simulink model "playground"  (R2024a)
settings: Solver=ode45  StartTime=0.0  StopTime=10.0  FixedStep=0.001  RelTol=1e-3
values from neighbouring files (symbols this model uses):
  a_r = 1.14 * 10^(-7)    (= 1.14e-07)    [start.m]    (also in startEnglPaper.m = 0.033; startReduced.m)
  a_rS = b    (= 0.033)    [startEnglPaper.m]
  A_x = 0.25    [playgrounMat.m]    (also in start.m; startEnglPaper.m; startReduced.m)
  A_y = 0.25    [playgrounMat.m]    (also in start.m; startEnglPaper.m; startReduced.m)
  A_z = 0.25    [playgrounMat.m]    (also in start.m; startEnglPaper.m; startReduced.m)
  b = 1.14 * 10^(-7)    (= 1.14e-07)    [start.m]    (also in startEnglPaper.m = 0.033; startReduced.m)
  g = 9.81    [playgrounMat.m]    (also in start.m; startEnglPaper.m; startReduced.m)
  gamma_d = pi/3    (= 1.0471975512)    [start.m]    (also in startReduced.m)
  I_r = 5.38 * 10 ^ (-5)    (= 5.38e-05)    [start.m]    (also in startEnglPaper.m = 3.38e-05; startReduced.m)
  I_x = 0.0151    [start.m]    (also in startEnglPaper.m = 0.004856; startReduced.m)
  I_y = 0.253    [start.m]    (also in startEnglPaper.m = 0.004856; startReduced.m)
  I_z = 0.0151    [start.m]    (also in startEnglPaper.m = 0.008801; startReduced.m)
  IrS = 5.38 * 10^(-5)    (= 5.38e-05)    [startEnglPaper.m]
  IxS = 0.0151    [startEnglPaper.m]
  IyS = IxS    (= 0.0151)    [startEnglPaper.m]
  IzS = 0.0253    [startEnglPaper.m]
  k = 1.045 * 10^(-11)    (= 1.045e-11)    [start.m]    (also in startEnglPaper.m = 2.98e-06; startReduced.m)
  K_gamma_D1 = K(1)    [playgrounMat.m]
  K_gamma_I1 = K(3)    [playgrounMat.m]
  K_gamma_P1 = K(2)    [playgrounMat.m]
  K_phi_D1 = 0.047    [startEnglPaper.m]
  K_phi_D11 = 0.093    [startEnglPaper.m]
  K_phi_D2 = 9.6    [startEnglPaper.m]
  K_phi_D22 = 19.2    [startEnglPaper.m]
  K_phi_DS = 0.14    [startEnglPaper.m]
  K_phi_I11 = 1.27    [startEnglPaper.m]
  K_phi_I22 = 262.144    [startEnglPaper.m]
  K_phi_P1 = 0.11    [startEnglPaper.m]
  K_phi_P11 = 0.5966    [startEnglPaper.m]
  K_phi_P2 = 23.04    [startEnglPaper.m]
  K_phi_P22 = 122.88    [startEnglPaper.m]
  K_phi_PS = 0.35    [startEnglPaper.m]
  K_psi_D = 40    [start.m]    (also in startEnglPaper.m = 9.6; startReduced.m)
  K_psi_D1 = 0.0844    [startEnglPaper.m]
  K_psi_D2 = 9.6    [startEnglPaper.m]
  K_psi_D22 = 19.2    [startEnglPaper.m]
  K_psi_DS = 0.24    [startEnglPaper.m]
  K_psi_I22 = 262.144    [startEnglPaper.m]
  K_psi_P = 143    [start.m]    (also in startEnglPaper.m = 23.04; startReduced.m)
  K_psi_P1 = 0.202    [startEnglPaper.m]
  K_psi_P2 = 23.04    [startEnglPaper.m]
  K_psi_P22 = 122.88    [startEnglPaper.m]
  K_psi_PS = 0.58    [startEnglPaper.m]
  K_theta_D = 58    [start.m]    (also in startEnglPaper.m = 9.6; startReduced.m)
  K_theta_D1 = 0.047    [startEnglPaper.m]
  K_theta_D2 = 9.6    [startEnglPaper.m]
  K_theta_D22 = 19.2    [startEnglPaper.m]
  K_theta_DS = 0.14    [startEnglPaper.m]
  K_theta_I22 = 262.144    [startEnglPaper.m]
  K_theta_P = 141    [start.m]    (also in startEnglPaper.m = 23.04; startReduced.m)
  K_theta_P1 = 0.11    [startEnglPaper.m]
  K_theta_P2 = 23.04    [startEnglPaper.m]
  K_theta_P22 = 122.88    [startEnglPaper.m]
  K_theta_PS = 0.35    [startEnglPaper.m]
  K_y_D = 13.58    [start.m]    (also in startReduced.m)
  K_y_P = 33.18    [start.m]    (also in startReduced.m)
  K_z_D1 = 4.42    [startEnglPaper.m]
  K_z_D2 = 4.42/m + A_z/m    (= 9.60905349794)    [startEnglPaper.m]
  K_z_DS = 13.58    [startEnglPaper.m]
  K_z_P1 = 11.2    [startEnglPaper.m]
  K_z_P2 = 11.2/m + A_z/m    (= 23.5596707819)    [startEnglPaper.m]
  K_z_PS = 33.18    [startEnglPaper.m]
  kl = 3 * 10^(-6)    (= 3e-06)    [startEnglPaper.m]
  l = 0.225    [start.m]    (also in startEnglPaper.m; startReduced.m)
  m = 1.44    [playgrounMat.m]    (also in start.m; startEnglPaper.m = 0.486; startReduced.m)
  m_s = [1/4 0 -1/(2*l) -1/(4*a_r); 1/4 -1/(2*l) 0 1/(4*a_r); 1/4 0 1/(2*l) -1/(4*a_r); 1/4 1/(2*l) 0 1/(4*a_r)]    [start.m]    (also in startReduced.m)
  mS = 1.44    [startEnglPaper.m]
  phi_d = 0.2    [startEnglPaper.m]
  phi_DesS = 0.2    [startEnglPaper.m]
  phi_init = 0    [startEnglPaper.m]
  phi_iS = 0;   deg2rad(10)    [startEnglPaper.m]
  psi_d = pi/5    (= 0.628318530718)    [start.m]    (also in startEnglPaper.m = 0.15; startReduced.m)
  psi_DesS = 0.15    [startEnglPaper.m]
  psi_init = 0    [startEnglPaper.m]
  psi_iS = 0    [startEnglPaper.m]
  theta_d = pi/4    (= 0.785398163397)    [start.m]    (also in startEnglPaper.m = 0.3; startReduced.m)
  theta_DesS = -0.1 * -3    (= 0.3)    [startEnglPaper.m]
  theta_init = 0    [startEnglPaper.m]
  theta_iS = 0    [startEnglPaper.m]
  x_init = 0    [startEnglPaper.m]
  x_iS = 0    [startEnglPaper.m]
  y_init = 0    [startEnglPaper.m]
  y_iS = 0    [startEnglPaper.m]
  z_d = 0.05 * 0    (= 0)    [startEnglPaper.m]
  z_DesS = 0.1    [startEnglPaper.m]
  z_init = 0    [startEnglPaper.m]
  z_iS = 0.0    (= 0)    [startEnglPaper.m]
undefined symbols (not defined in the file or in its folder): m_s_my
libraries: slpidlib x14
(part 1 of 4)
settings Model: Creator=Илья  LastModifiedBy=Илья

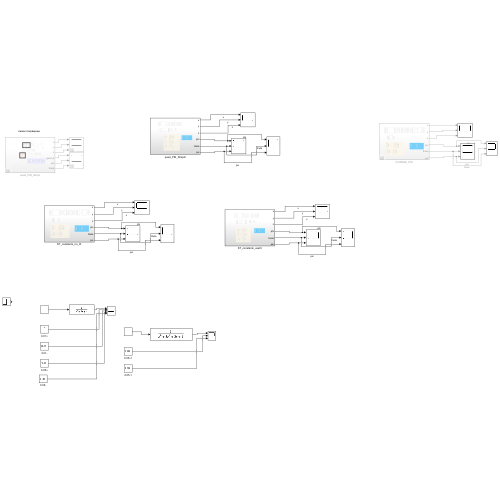
[thumbnail: Simulink's stored preview of the top-level diagram]
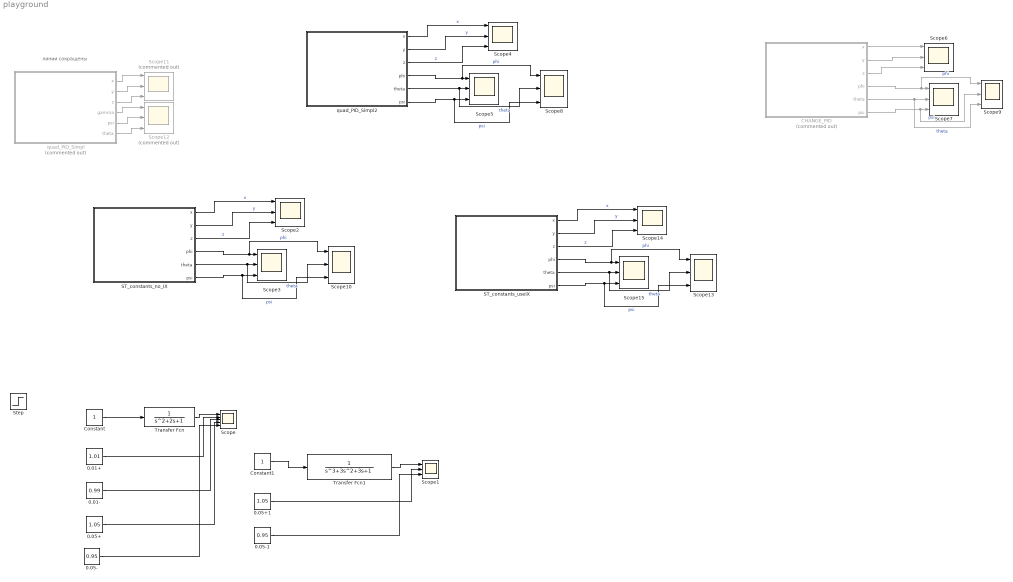
== system playground ==
  note: линии сокращены
  0.01+ : Constant  Value=1.01
  0.01- : Constant  Value=0.99
  0.05+ : Constant  Value=1.05
  0.05+1 : Constant  Value=1.05
  0.05- : Constant  Value=0.95
  0.05-1 : Constant  Value=0.95
  CHANGE_PID : Subsystem  Commented=on
  Constant : Constant
  Constant1 : Constant
  ST_constants_no_IX : Subsystem
  ST_constants_useIX : Subsystem
  Scope : Scope  NumInputPorts=5
  Scope{1..10,13..15} (13 alike) : Scope  NumInputPorts=3
  Scope11 : Scope  Commented=on  NumInputPorts=3
  Scope12 : Scope  Commented=on  NumInputPorts=3
  Step : Step  SampleTime=0
  Transfer Fcn : TransferFcn
  Transfer Fcn1 : TransferFcn  Denominator=[1 3 3 1]
  quad_PID_Simpl : Subsystem  Commented=on
  quad_PID_Simpl2 : Subsystem
  wires:
  Transfer Fcn/1 -> Scope/1
  Constant/1 -> Transfer Fcn/1
  0.01+/1 -> Scope/2
  0.01-/1 -> Scope/3
  0.05+/1 -> Scope/4
  0.05-/1 -> Scope/5
  Constant1/1 -> Transfer Fcn1/1
  Transfer Fcn1/1 -> Scope1/1
  0.05+1/1 -> Scope1/2
  0.05-1/1 -> Scope1/3
  quad_PID_Simpl/5(psi) -> Scope12/2
  quad_PID_Simpl/3(z) -> Scope11/3
  quad_PID_Simpl/4(gamma) -> Scope12/1
  quad_PID_Simpl/1(x) -> Scope11/1
  quad_PID_Simpl/2(y) -> Scope11/2
  quad_PID_Simpl/6(theta) -> Scope12/3
  quad_PID_Simpl2/2(y) -> Scope4/2  "y"
  quad_PID_Simpl2/3(z) -> Scope4/3  "z"
  quad_PID_Simpl2/6(psi) -> Scope8/3, Scope5/3  "psi"
  quad_PID_Simpl2/4(phi) -> Scope8/1, Scope5/1  "phi"
  quad_PID_Simpl2/5(theta) -> Scope8/2, Scope5/2  "theta"
  quad_PID_Simpl2/1(x) -> Scope4/1  "x"
  CHANGE_PID/1(x) -> Scope6/1
  CHANGE_PID/5(theta) -> Scope9/3, Scope7/2  "theta"
  CHANGE_PID/4(phi) -> Scope9/1, Scope7/1  "phi"
  CHANGE_PID/6(psi) -> Scope9/2, Scope7/3  "psi"
  CHANGE_PID/3(z) -> Scope6/3
  CHANGE_PID/2(y) -> Scope6/2
  ST_constants_no_IX/1(x) -> Scope2/1  "x"
  ST_constants_no_IX/5(theta) -> Scope3/2, Scope10/2  "theta"
  ST_constants_no_IX/4(phi) -> Scope3/1, Scope10/1  "phi"
  ST_constants_no_IX/6(psi) -> Scope3/3, Scope10/3  "psi"
  ST_constants_no_IX/3(z) -> Scope2/3  "z"
  ST_constants_no_IX/2(y) -> Scope2/2  "y"
  ST_constants_useIX/2(y) -> Scope14/2  "y"
  ST_constants_useIX/3(z) -> Scope14/3  "z"
  ST_constants_useIX/6(psi) -> Scope13/3, Scope15/3  "psi"
  ST_constants_useIX/4(phi) -> Scope13/1, Scope15/1  "phi"
  ST_constants_useIX/5(theta) -> Scope13/2, Scope15/2  "theta"
  ST_constants_useIX/1(x) -> Scope14/1  "x"

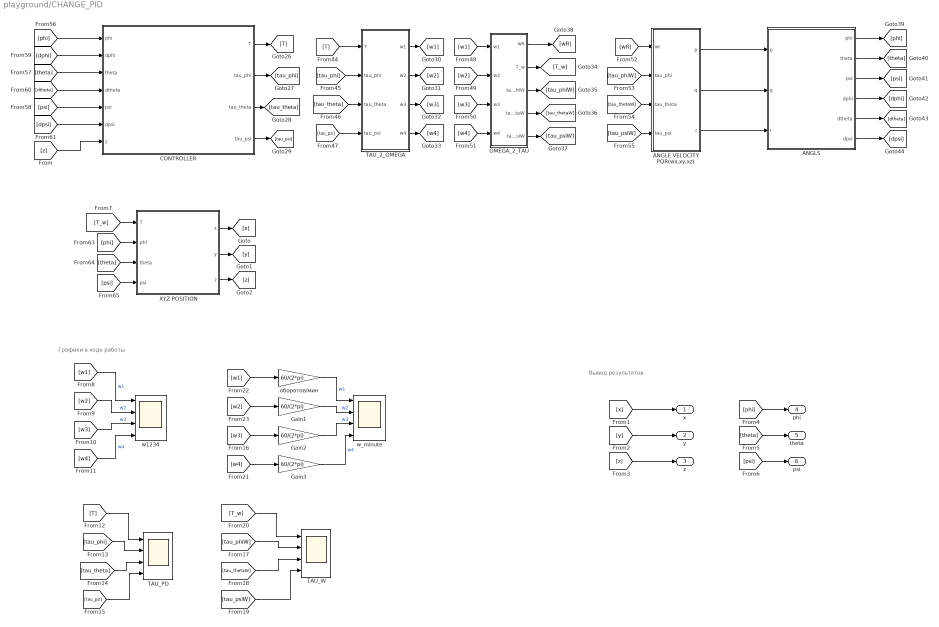
== system playground/CHANGE_PID ==
  note: Графики в ходе работы
  note: Вывод результатов
  ANGLE VELOCITY PQR(wx,xy,xz) : Subsystem
  ANGLS : Subsystem
  CONTROLLER : Subsystem
  Gain1 : Gain  Gain=60/(2*pi)
  Gain2 : Gain  Gain=60/(2*pi)
  Gain3 : Gain  Gain=60/(2*pi)
  OMEGA_2_TAU : Subsystem
  TAU_2_OMEGA : Subsystem
  TAU_PD : Scope  NumInputPorts=4
  TAU_W : Scope  NumInputPorts=4
  XYZ POSITION : Subsystem
  w1234 : Scope  NumInputPorts=4
  w_minute : Scope  NumInputPorts=4
  оборотов/мин : Gain  Gain=60/(2*pi)
  x : Outport
  y : Outport  Port=2
  z : Outport  Port=3
  phi : Outport  Port=4
  theta : Outport  Port=5
  psi : Outport  Port=6
  wires:
  Gain3/1 -> w_minute/4  "w4"
  Gain2/1 -> w_minute/3  "w3"
  Gain1/1 -> w_minute/2  "w2"
  оборотов/мин/1 -> w_minute/1  "w1"
  [w4] -> Gain3/1
  [w3] -> Gain2/1
  [w2] -> Gain1/1
  [w1] -> оборотов/мин/1
  [tau_psiW] -> TAU_W/4
  [tau_thetaW] -> TAU_W/3
  [tau_phiW] -> TAU_W/2
  [T_w] -> TAU_W/1
  [tau_psi] -> TAU_PD/4
  [tau_theta] -> TAU_PD/3
  [tau_phi] -> TAU_PD/2
  [T] -> TAU_PD/1
  [w4] -> w1234/4  "w4"
  [w3] -> w1234/3  "w3"
  [w2] -> w1234/2  "w2"
  [w1] -> w1234/1  "w1"
  [psi] -> psi/1
  [theta] -> theta/1
  [phi] -> phi/1
  [z] -> z/1
  [y] -> y/1
  [x] -> x/1
  [z] -> CONTROLLER/7(z)
  XYZ POSITION/3(z) -> [z]
  XYZ POSITION/2(y) -> [y]
  XYZ POSITION/1(x) -> [x]
  [psi] -> XYZ POSITION/4(psi)
  [theta] -> XYZ POSITION/3(theta)
  [phi] -> XYZ POSITION/2(phi)
  [T_w] -> XYZ POSITION/1(T)
  [psi] -> CONTROLLER/5(psi)
  [dpsi] -> CONTROLLER/6(dpsi)
  [dtheta] -> CONTROLLER/4(dtheta)
  [theta] -> CONTROLLER/3(theta)
  [dphi] -> CONTROLLER/2(dphi)
  [phi] -> CONTROLLER/1(phi)
  ANGLE VELOCITY PQR(wx,xy,xz)/3(r) -> ANGLS/3(r)
  ANGLE VELOCITY PQR(wx,xy,xz)/2(q) -> ANGLS/2(q)
  ANGLE VELOCITY PQR(wx,xy,xz)/1(p) -> ANGLS/1(p)
  ANGLS/6(dpsi) -> [dpsi]
  ANGLS/5(dtheta) -> [dtheta]
  ANGLS/4(dphi) -> [dphi]
  ANGLS/3(psi) -> [psi]
  ANGLS/2(theta) -> [theta]
  ANGLS/1(phi) -> [phi]
  [tau_psiW] -> ANGLE VELOCITY PQR(wx,xy,xz)/4(tau_psi)
  [tau_thetaW] -> ANGLE VELOCITY PQR(wx,xy,xz)/3(tau_theta)
  [tau_phiW] -> ANGLE VELOCITY PQR(wx,xy,xz)/2(tau_phi)
  [wR] -> ANGLE VELOCITY PQR(wx,xy,xz)/1(wr)
  OMEGA_2_TAU/1(wR) -> [wR]
  OMEGA_2_TAU/5(tau_psiW) -> [tau_psiW]
  OMEGA_2_TAU/4(tau_thetaW) -> [tau_thetaW]
  OMEGA_2_TAU/3(tau_phiW) -> [tau_phiW]
  OMEGA_2_TAU/2(T_w) -> [T_w]
  [w4] -> OMEGA_2_TAU/4(w4)
  [w3] -> OMEGA_2_TAU/3(w3)
  [w2] -> OMEGA_2_TAU/2(w2)
  [w1] -> OMEGA_2_TAU/1(w1)
  TAU_2_OMEGA/4(w4) -> [w4]
  TAU_2_OMEGA/3(w3) -> [w3]
  TAU_2_OMEGA/2(w2) -> [w2]
  TAU_2_OMEGA/1(w1) -> [w1]
  [tau_psi] -> TAU_2_OMEGA/4(tau_psi)
  [tau_theta] -> TAU_2_OMEGA/3(tau_theta)
  [tau_phi] -> TAU_2_OMEGA/2(tau_phi)
  [T] -> TAU_2_OMEGA/1(T)
  CONTROLLER/4(tau_psi) -> [tau_psi]
  CONTROLLER/3(tau_theta) -> [tau_theta]
  CONTROLLER/2(tau_phi) -> [tau_phi]
  CONTROLLER/1(T) -> [T]

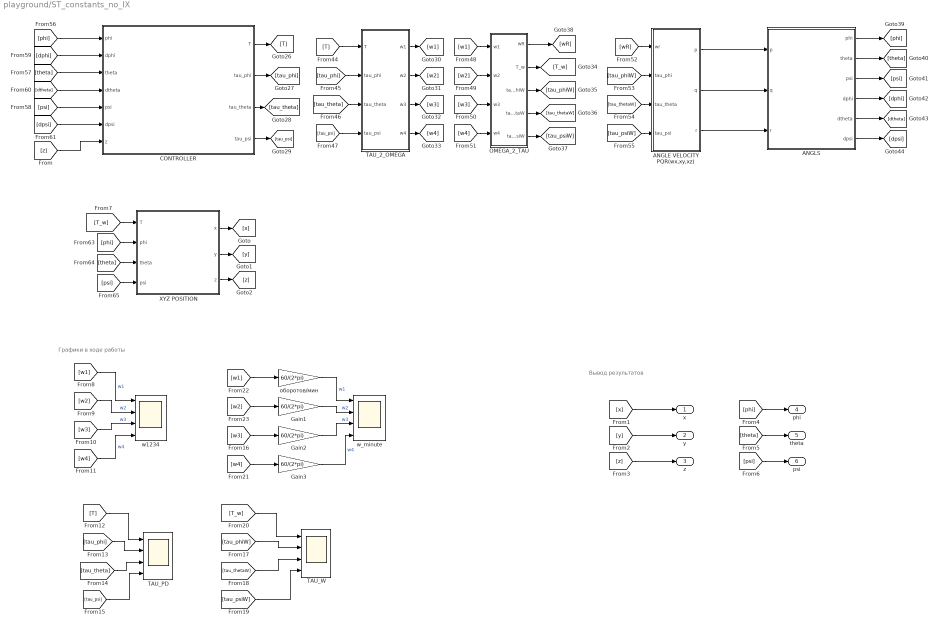
== system playground/ST_constants_no_IX ==
  note: Графики в ходе работы
  note: Вывод результатов
  ANGLE VELOCITY PQR(wx,xy,xz) : Subsystem
  ANGLS : Subsystem
  CONTROLLER : Subsystem
  Gain1 : Gain  Gain=60/(2*pi)
  Gain2 : Gain  Gain=60/(2*pi)
  Gain3 : Gain  Gain=60/(2*pi)
  OMEGA_2_TAU : Subsystem
  TAU_2_OMEGA : Subsystem
  TAU_PD : Scope  NumInputPorts=4
  TAU_W : Scope  NumInputPorts=4
  XYZ POSITION : Subsystem
  w1234 : Scope  NumInputPorts=4
  w_minute : Scope  NumInputPorts=4
  оборотов/мин : Gain  Gain=60/(2*pi)
  x : Outport
  y : Outport  Port=2
  z : Outport  Port=3
  phi : Outport  Port=4
  theta : Outport  Port=5
  psi : Outport  Port=6
  wires:
  Gain3/1 -> w_minute/4  "w4"
  Gain2/1 -> w_minute/3  "w3"
  Gain1/1 -> w_minute/2  "w2"
  оборотов/мин/1 -> w_minute/1  "w1"
  [w4] -> Gain3/1
  [w3] -> Gain2/1
  [w2] -> Gain1/1
  [w1] -> оборотов/мин/1
  [tau_psiW] -> TAU_W/4
  [tau_thetaW] -> TAU_W/3
  [tau_phiW] -> TAU_W/2
  [T_w] -> TAU_W/1
  [tau_psi] -> TAU_PD/4
  [tau_theta] -> TAU_PD/3
  [tau_phi] -> TAU_PD/2
  [T] -> TAU_PD/1
  [w4] -> w1234/4  "w4"
  [w3] -> w1234/3  "w3"
  [w2] -> w1234/2  "w2"
  [w1] -> w1234/1  "w1"
  [psi] -> psi/1
  [theta] -> theta/1
  [phi] -> phi/1
  [z] -> z/1
  [y] -> y/1
  [x] -> x/1
  [z] -> CONTROLLER/7(z)
  XYZ POSITION/3(z) -> [z]
  XYZ POSITION/2(y) -> [y]
  XYZ POSITION/1(x) -> [x]
  [psi] -> XYZ POSITION/4(psi)
  [theta] -> XYZ POSITION/3(theta)
  [phi] -> XYZ POSITION/2(phi)
  [T_w] -> XYZ POSITION/1(T)
  [psi] -> CONTROLLER/5(psi)
  [dpsi] -> CONTROLLER/6(dpsi)
  [dtheta] -> CONTROLLER/4(dtheta)
  [theta] -> CONTROLLER/3(theta)
  [dphi] -> CONTROLLER/2(dphi)
  [phi] -> CONTROLLER/1(phi)
  ANGLE VELOCITY PQR(wx,xy,xz)/3(r) -> ANGLS/3(r)
  ANGLE VELOCITY PQR(wx,xy,xz)/2(q) -> ANGLS/2(q)
  ANGLE VELOCITY PQR(wx,xy,xz)/1(p) -> ANGLS/1(p)
  ANGLS/6(dpsi) -> [dpsi]
  ANGLS/5(dtheta) -> [dtheta]
  ANGLS/4(dphi) -> [dphi]
  ANGLS/3(psi) -> [psi]
  ANGLS/2(theta) -> [theta]
  ANGLS/1(phi) -> [phi]
  [tau_psiW] -> ANGLE VELOCITY PQR(wx,xy,xz)/4(tau_psi)
  [tau_thetaW] -> ANGLE VELOCITY PQR(wx,xy,xz)/3(tau_theta)
  [tau_phiW] -> ANGLE VELOCITY PQR(wx,xy,xz)/2(tau_phi)
  [wR] -> ANGLE VELOCITY PQR(wx,xy,xz)/1(wr)
  OMEGA_2_TAU/1(wR) -> [wR]
  OMEGA_2_TAU/5(tau_psiW) -> [tau_psiW]
  OMEGA_2_TAU/4(tau_thetaW) -> [tau_thetaW]
  OMEGA_2_TAU/3(tau_phiW) -> [tau_phiW]
  OMEGA_2_TAU/2(T_w) -> [T_w]
  [w4] -> OMEGA_2_TAU/4(w4)
  [w3] -> OMEGA_2_TAU/3(w3)
  [w2] -> OMEGA_2_TAU/2(w2)
  [w1] -> OMEGA_2_TAU/1(w1)
  TAU_2_OMEGA/4(w4) -> [w4]
  TAU_2_OMEGA/3(w3) -> [w3]
  TAU_2_OMEGA/2(w2) -> [w2]
  TAU_2_OMEGA/1(w1) -> [w1]
  [tau_psi] -> TAU_2_OMEGA/4(tau_psi)
  [tau_theta] -> TAU_2_OMEGA/3(tau_theta)
  [tau_phi] -> TAU_2_OMEGA/2(tau_phi)
  [T] -> TAU_2_OMEGA/1(T)
  CONTROLLER/4(tau_psi) -> [tau_psi]
  CONTROLLER/3(tau_theta) -> [tau_theta]
  CONTROLLER/2(tau_phi) -> [tau_phi]
  CONTROLLER/1(T) -> [T]

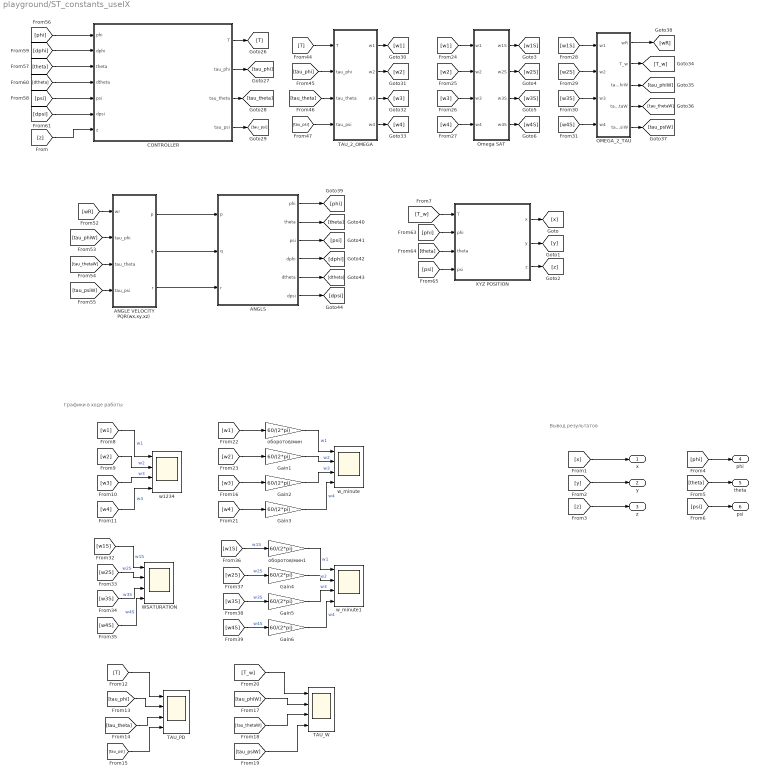
== system playground/ST_constants_useIX ==
  note: Вывод результатов
  note: Графики в ходе работы
  ANGLE VELOCITY PQR(wx,xy,xz) : Subsystem
  ANGLS : Subsystem
  CONTROLLER : Subsystem
  Gain{1..6} (6 alike) : Gain  Gain=60/(2*pi)
  OMEGA_2_TAU : Subsystem
  Omega SAT : Subsystem
  TAU_2_OMEGA : Subsystem
  TAU_PD : Scope  NumInputPorts=4
  TAU_W : Scope  NumInputPorts=4
  WSATURATION : Scope  NumInputPorts=4
  XYZ POSITION : Subsystem
  w1234 : Scope  NumInputPorts=4
  w_minute : Scope  NumInputPorts=4
  w_minute1 : Scope  NumInputPorts=4
  оборотов/мин : Gain  Gain=60/(2*pi)
  оборотов/мин1 : Gain  Gain=60/(2*pi)
  x : Outport
  y : Outport  Port=2
  z : Outport  Port=3
  phi : Outport  Port=4
  theta : Outport  Port=5
  psi : Outport  Port=6
  wires:
  CONTROLLER/1(T) -> [T]
  CONTROLLER/2(tau_phi) -> [tau_phi]
  CONTROLLER/3(tau_theta) -> [tau_theta]
  CONTROLLER/4(tau_psi) -> [tau_psi]
  [T] -> TAU_2_OMEGA/1(T)
  [tau_phi] -> TAU_2_OMEGA/2(tau_phi)
  [tau_theta] -> TAU_2_OMEGA/3(tau_theta)
  [tau_psi] -> TAU_2_OMEGA/4(tau_psi)
  TAU_2_OMEGA/1(w1) -> [w1]
  TAU_2_OMEGA/2(w2) -> [w2]
  TAU_2_OMEGA/3(w3) -> [w3]
  TAU_2_OMEGA/4(w4) -> [w4]
  [w1S] -> OMEGA_2_TAU/1(w1)
  [w2S] -> OMEGA_2_TAU/2(w2)
  [w3S] -> OMEGA_2_TAU/3(w3)
  [w4S] -> OMEGA_2_TAU/4(w4)
  OMEGA_2_TAU/2(T_w) -> [T_w]
  OMEGA_2_TAU/3(tau_phiW) -> [tau_phiW]
  OMEGA_2_TAU/4(tau_thetaW) -> [tau_thetaW]
  OMEGA_2_TAU/5(tau_psiW) -> [tau_psiW]
  OMEGA_2_TAU/1(wR) -> [wR]
  [wR] -> ANGLE VELOCITY PQR(wx,xy,xz)/1(wr)
  [tau_phiW] -> ANGLE VELOCITY PQR(wx,xy,xz)/2(tau_phi)
  [tau_thetaW] -> ANGLE VELOCITY PQR(wx,xy,xz)/3(tau_theta)
  [tau_psiW] -> ANGLE VELOCITY PQR(wx,xy,xz)/4(tau_psi)
  ANGLS/1(phi) -> [phi]
  ANGLS/2(theta) -> [theta]
  ANGLS/3(psi) -> [psi]
  ANGLS/4(dphi) -> [dphi]
  ANGLS/5(dtheta) -> [dtheta]
  ANGLS/6(dpsi) -> [dpsi]
  ANGLE VELOCITY PQR(wx,xy,xz)/1(p) -> ANGLS/1(p)
  ANGLE VELOCITY PQR(wx,xy,xz)/2(q) -> ANGLS/2(q)
  ANGLE VELOCITY PQR(wx,xy,xz)/3(r) -> ANGLS/3(r)
  [phi] -> CONTROLLER/1(phi)
  [dphi] -> CONTROLLER/2(dphi)
  [theta] -> CONTROLLER/3(theta)
  [dtheta] -> CONTROLLER/4(dtheta)
  [dpsi] -> CONTROLLER/6(dpsi)
  [psi] -> CONTROLLER/5(psi)
  [T_w] -> XYZ POSITION/1(T)
  [phi] -> XYZ POSITION/2(phi)
  [theta] -> XYZ POSITION/3(theta)
  [psi] -> XYZ POSITION/4(psi)
  XYZ POSITION/1(x) -> [x]
  XYZ POSITION/2(y) -> [y]
  XYZ POSITION/3(z) -> [z]
  [z] -> CONTROLLER/7(z)
  [x] -> x/1
  [y] -> y/1
  [z] -> z/1
  [phi] -> phi/1
  [theta] -> theta/1
  [psi] -> psi/1
  [w1] -> w1234/1  "w1"
  [w2] -> w1234/2  "w2"
  [w3] -> w1234/3  "w3"
  [w4] -> w1234/4  "w4"
  [T] -> TAU_PD/1
  [tau_phi] -> TAU_PD/2
  [tau_theta] -> TAU_PD/3
  [tau_psi] -> TAU_PD/4
  [T_w] -> TAU_W/1
  [tau_phiW] -> TAU_W/2
  [tau_thetaW] -> TAU_W/3
  [tau_psiW] -> TAU_W/4
  [w1] -> оборотов/мин/1
  [w2] -> Gain1/1
  [w3] -> Gain2/1
  [w4] -> Gain3/1
  оборотов/мин/1 -> w_minute/1  "w1"
  Gain1/1 -> w_minute/2  "w2"
  Gain2/1 -> w_minute/3  "w3"
  Gain3/1 -> w_minute/4  "w4"
  [w4] -> Omega SAT/4(w4)
  Omega SAT/2(w2S) -> [w2S]
  [w1] -> Omega SAT/1(w1)
  [w3] -> Omega SAT/3(w3)
  Omega SAT/4(w4S) -> [w4S]
  Omega SAT/1(w1S) -> [w1S]
  Omega SAT/3(w3S) -> [w3S]
  [w2] -> Omega SAT/2(w2)
  [w3S] -> Gain5/1  "w3S"
  Gain5/1 -> w_minute1/3  "w3"
  оборотов/мин1/1 -> w_minute1/1  "w1"
  [w4S] -> WSATURATION/4  "w4S"
  [w4S] -> Gain6/1  "w4S"
  [w1S] -> оборотов/мин1/1  "w1S"
  Gain6/1 -> w_minute1/4  "w4"
  Gain4/1 -> w_minute1/2  "w2"
  [w2S] -> WSATURATION/2  "w2S"
  [w3S] -> WSATURATION/3  "w3S"
  [w1S] -> WSATURATION/1  "w1S"
  [w2S] -> Gain4/1  "w2S"

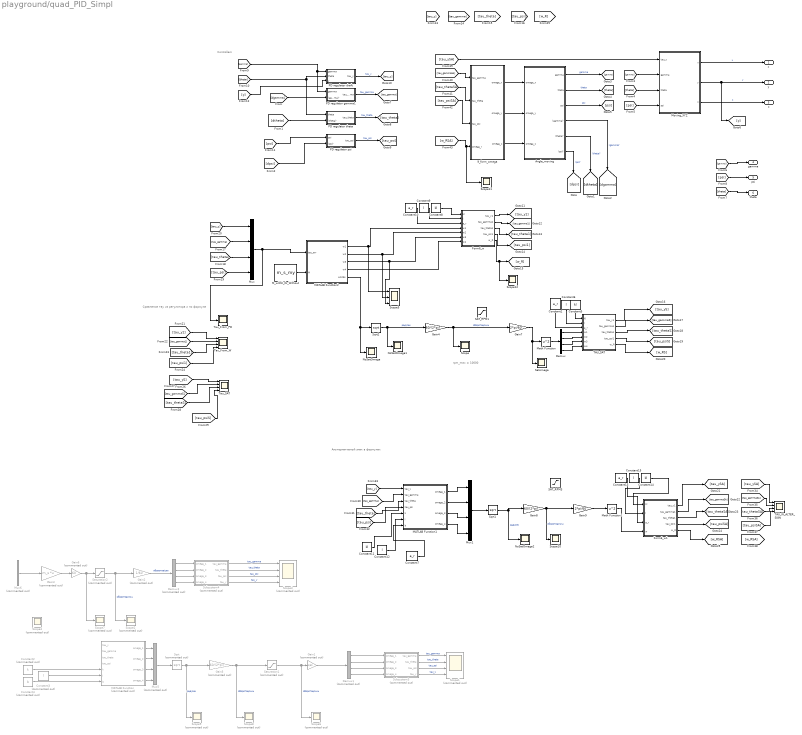
== system playground/quad_PID_Simpl ==
  note: Сравнение тау из регулятора и по формуле
  note: Controllers
  note: rpm_max = 10000
  note: Альтернативный знак в формулах
  9_form_omega : Subsystem
  Angle_moving : Subsystem
  Constant{1,7,10,13} (4 alike) : Constant  Value=a_r
  Constant{5,8,11,14} (4 alike) : Constant  Value=kl
  Constant{6,9,12,15} (4 alike) : Constant  Value=l
  Constant2 : Constant  Commented=on  Value=k
  Constant3 : Constant  Commented=on  Value=l
  Constant4 : Constant  Commented=on  Value=b
  Demux : Demux
  Demux1 : Demux  Commented=on
  Demux2 : Demux  Commented=on
  Form6_w : MATLAB Function  TreatAsAtomicUnit=on
  Form6_w1 : MATLAB Function  TreatAsAtomicUnit=on
  Gain1 : Gain  Commented=on  Gain=1/60
  Gain2 : Gain  Commented=on  Gain=1/60
  Gain3 : Gain  Commented=on  Gain=m_s  Multiplication=Matrix(K*u) (u vector)
  Gain4 : Gain  Gain=60/(2*pi)
  Gain5 : Gain  Commented=on  Gain=60/(2*pi)
  Gain6 : Gain  Commented=on  Gain=60
  Gain7 : Gain  Gain=2*pi/60
  Gain8 : Gain  Gain=60/(2*pi)
  Gain9 : Gain  Gain=2*pi/60
  MATLAB Function : MATLAB Function  Commented=on  TreatAsAtomicUnit=on
  MATLAB Function1 : MATLAB Function  TreatAsAtomicUnit=on
  MATLAB Function2 : MATLAB Function  TreatAsAtomicUnit=on
  M_withK_Or_Without : Constant  Value=m_s_my
  Math Function : Math  Operator=square  SignedPower=on
  Math Function1 : Math  Operator=square  SignedPower=on
  Moving_XYZ : Subsystem
  Mux : Mux
  Mux1 : Mux
  Mux5 : Mux  Commented=on
  Mux6 : Mux  Commented=on
  NoSatOmega : Scope
  NoSatOmega1 : Scope
  NoSatOmega2 : Scope
  PD regulator draft : Subsystem
  PD regulator gamma1 : Subsystem
  PD regulator psi : Subsystem
  PD regulator theta : Subsystem
  SAT_RPM1 : Saturate  UpperLimit=20000  LowerLimit=1500
  SAT_RPM3 : Saturate  UpperLimit=14000  LowerLimit=1500
  Satomega : Scope
  Saturation1 : Saturate  Commented=on  UpperLimit=15000  LowerLimit=1000
  Saturation2 : Saturate  Commented=on  UpperLimit=15000  LowerLimit=1000
  Scope{,10..12} (4 alike) : Scope
  Scope1 : Scope  Commented=on  NumInputPorts=4
  Scope{2,4,6..9} (6 alike) : Scope  Commented=on
  Scope3 : Scope  Commented=on  NumInputPorts=4
  Scope5 : Scope  NumInputPorts=3
  Sqrt : Sqrt  Commented=on
  Sqrt1 : Sqrt
  Sqrt2 : Sqrt
  Subsystem3 : Subsystem  Commented=on
  Subsystem4 : Subsystem  Commented=on
  TAU_SAT : MATLAB Function  TreatAsAtomicUnit=on
  TAU_W_ALTER_SIGN : Scope  NumInputPorts=4
  Tau_From_PD : Scope
  Tau_From_W : Scope  NumInputPorts=4
  Tau_SAT : Scope  NumInputPorts=4
  x : Outport
  y : Outport  Port=2
  z : Outport  Port=3
  gamma : Outport  Port=4
  psi : Outport  Port=5
  theta : Outport  Port=6
  wires:
  Form6_w/5(w_R) -> Scope12/1, [w_R]
  Gain4/1 -> Gain7/1, Scope/1  "оборотов/мин"
  Sqrt2/1 -> NoSatOmega1/1, Gain4/1  "рад/сек"
  Constant10/1 -> Form6_w/3(a_r)
  Constant9/1 -> Form6_w/2(l)
  Constant8/1 -> Form6_w/1(kl)
  MATLAB Function2/4(w4) -> Form6_w/7(w4)
  MATLAB Function2/3(w3) -> Scope5/3, Form6_w/6(w3)
  MATLAB Function2/2(w2) -> Scope5/2, Form6_w/5(w2)
  MATLAB Function2/1(w1) -> Scope5/1, Form6_w/4(w1)
  [tau_psi1] -> Tau_From_W/4
  [tau_theta1] -> Tau_From_W/3
  [tau_gamma1] -> Tau_From_W/2
  [tau_y1] -> Tau_From_W/1
  Form6_w/4(tau_psi1) -> [tau_psi1]
  Form6_w/3(tau_theta1) -> [tau_theta1]
  Form6_w/2(tau_gamma1) -> [tau_gamma1]
  Form6_w/1(tau_y1) -> [tau_y1]
  MATLAB Function2/5(w1234) -> Sqrt2/1, NoSatOmega/1
  M_withK_Or_Without/1 -> MATLAB Function2/2(M)
  Mux/1 -> MATLAB Function2/1(tau_arr), Tau_From_PD/1
  [tau_psi] -> Mux/4
  [tau_theta] -> Mux/3
  [tau_gamma] -> Mux/2
  [tau_y] -> Mux/1
  [theta] -> theta/1
  [psi] -> psi/1
  [y] -> PD regulator draft/3(y)
  [psi] -> PD regulator psi/1(psi)
  [theta] -> PD regulator draft/2(theta), PD regulator theta/1(theta)
  [gamma] -> PD regulator gamma1/1(gamma), PD regulator draft/1(gamma)
  [gamma] -> gamma/1
  [psi] -> Moving_XYZ/4(psi)
  [theta] -> Moving_XYZ/3(theta)
  [gamma] -> Moving_XYZ/2(gamma)
  [dpsi] -> PD regulator psi/2((psi)')
  [dtheta] -> PD regulator theta/2((theta)')
  [dgamma] -> PD regulator gamma1/2((gamma)')
  Angle_moving/1(gamma) -> [gamma]  "gamma"
  9_form_omega/2(omega_y) -> Angle_moving/2(omega_y)
  9_form_omega/3(omega_z) -> Angle_moving/3(omega_z)
  Angle_moving/5((theta)') -> [dtheta]  "(theta)'"
  9_form_omega/1(omega_x) -> Angle_moving/1(omega_x)
  Moving_XYZ/1(x) -> x/1  "x"
  Moving_XYZ/2(y) -> [y], y/1  "y"
  Angle_moving/4((gamma)') -> [dgamma]  "(gamma)'"
  Angle_moving/3(psi) -> [psi]  "psi"
  Angle_moving/6((psi)') -> [dpsi]  "(psi)'"
  Angle_moving/2(theta) -> [theta]  "theta"
  Moving_XYZ/3(z) -> z/1  "z"
  Subsystem3/2(tau_theta) -> Scope1/2  "tau_theta"
  Subsystem3/3(tau_psi) -> Scope1/3  "tau_psi"
  Subsystem3/1(tau_gamma) -> Scope1/1  "tau_gamma"
  Constant2/1 -> MATLAB Function/5(k)
  Constant3/1 -> MATLAB Function/6(l)
  Constant4/1 -> MATLAB Function/7(b)
  MATLAB Function/1(omega_1) -> Mux5/1
  MATLAB Function/2(omega_2) -> Mux5/2
  MATLAB Function/3(omega_3) -> Mux5/3
  MATLAB Function/4(omega_4) -> Mux5/4
  Mux5/1 -> Sqrt/1
  Subsystem3/4(tau_y) -> Scope1/4  "tau_y"
  Mux6/1 -> Gain3/1
  Subsystem4/2(tau_theta) -> Scope3/2  "tau_theta"
  Subsystem4/3(tau_psi) -> Scope3/3  "tau_psi"
  Demux2/2 -> Subsystem4/2(omega_2)
  Demux2/1 -> Subsystem4/1(omega_1)
  Demux2/4 -> Subsystem4/4(omega_4)
  Demux2/3 -> Subsystem4/3(omega_3)
  Subsystem4/4(tau_y) -> Scope3/4  "tau_y"
  Subsystem4/1(tau_gamma) -> Scope3/1  "tau_gamma"
  Demux1/3 -> Subsystem3/3(omega_3)
  Demux1/4 -> Subsystem3/4(omega_4)
  Demux1/1 -> Subsystem3/1(omega_1)
  Demux1/2 -> Subsystem3/2(omega_2)
  Saturation2/1 -> Gain2/1, Scope2/1  "оборотов/мин"
  Gain6/1 -> Scope7/1, Saturation2/1
  Sqrt/1 -> Scope9/1, Gain5/1  "рад/сек"
  Saturation1/1 -> Gain1/1, Scope6/1  "оборотов/мин"
  Gain3/1 -> Gain6/1
  Gain5/1 -> Saturation1/1, Scope8/1  "оборотов/мин"
  Gain1/1 -> Demux1/1
  Gain2/1 -> Demux2/1  "оборотов/сек"
  PD regulator psi/1(tau_psi) -> [tau_psi]  "tau_psi"
  PD regulator theta/1(tau_theta) -> [tau_theta]  "tau_theta"
  PD regulator draft/1(tau_y) -> [tau_y]  "tau_y"
  PD regulator gamma1/1(tau_gamma) -> [tau_gamma]  "tau_gamma"
  Gain7/1 -> Satomega/1, Math Function/1
  Demux/1 -> TAU_SAT/4(w1)
  Demux/2 -> TAU_SAT/5(w2)
  Demux/3 -> TAU_SAT/6(w3)
  Demux/4 -> TAU_SAT/7(w4)
  Constant5/1 -> TAU_SAT/1(kl)
  Constant6/1 -> TAU_SAT/2(l)
  Constant1/1 -> TAU_SAT/3(a_r)
  TAU_SAT/1(tau_y1) -> [tau_yS]
  TAU_SAT/2(tau_gamma1) -> [tau_gammaS]
  TAU_SAT/3(tau_theta1) -> [tau_thetaS]
  TAU_SAT/4(tau_psi1) -> [tau_psiS]
  TAU_SAT/5(w_R) -> [w_RS]
  [tau_yS] -> Tau_SAT/1
  [tau_gammaS] -> Tau_SAT/2
  [tau_thetaS] -> Tau_SAT/3
  [tau_psiS] -> Tau_SAT/4
  Constant12/1 -> MATLAB Function1/6(l)
  Constant7/1 -> MATLAB Function1/7(b)
  Constant11/1 -> MATLAB Function1/5(k)
  [tau_y] -> MATLAB Function1/1(tau_y)
  [tau_gamma] -> MATLAB Function1/2(tau_gamma)
  [tau_theta] -> MATLAB Function1/3(tau_theta)
  [tau_psi] -> MATLAB Function1/4(tau_psi)
  MATLAB Function1/1(omega_1) -> Mux1/1
  MATLAB Function1/2(omega_2) -> Mux1/2
  MATLAB Function1/3(omega_3) -> Mux1/3
  MATLAB Function1/4(omega_4) -> Mux1/4
  Mux1/1 -> Sqrt1/1
  Sqrt1/1 -> Gain8/1, NoSatOmega2/1  "рад/сек"
  Math Function/1 -> Demux/1
  Constant14/1 -> Form6_w1/1(kl)
  Constant15/1 -> Form6_w1/2(l)
  Constant13/1 -> Form6_w1/3(a_r)
  Math Function1/1 -> Form6_w1/4(w)
  Gain8/1 -> Scope10/1, Gain9/1  "оборотов/мин"
  Gain9/1 -> Math Function1/1
  Form6_w1/1(tau_y1) -> [tau_ySA]
  Form6_w1/2(tau_gamma1) -> [tau_gammaSA]
  Form6_w1/3(tau_theta1) -> [tau_thetaSA]
  Form6_w1/4(tau_psi1) -> [tau_psiSA]
  Form6_w1/5(w_R) -> [w_RSA]
  [tau_ySA] -> TAU_W_ALTER_SIGN/1
  [tau_gammaSA] -> TAU_W_ALTER_SIGN/2
  [tau_thetaSA] -> TAU_W_ALTER_SIGN/3
  [tau_psiSA] -> TAU_W_ALTER_SIGN/4
  [tau_ySA] -> Moving_XYZ/1(tau_y)
  [tau_gammaSA] -> 9_form_omega/1(tau_gamma)
  [tau_thetaSA] -> 9_form_omega/2(tau_theta)
  [tau_psiSA] -> 9_form_omega/3(tau_psi)
  [w_RSA] -> Scope11/1, 9_form_omega/4(omega_r)

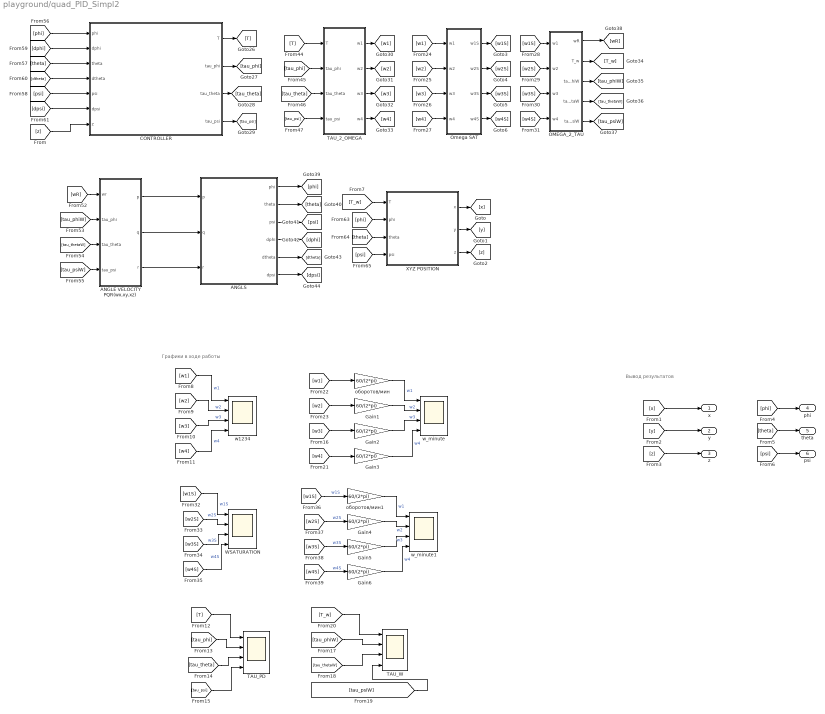
== system playground/quad_PID_Simpl2 ==
  note: Вывод результатов
  note: Графики в ходе работы
  ANGLE VELOCITY PQR(wx,xy,xz) : Subsystem
  ANGLS : Subsystem
  CONTROLLER : Subsystem
  Gain{1..6} (6 alike) : Gain  Gain=60/(2*pi)
  OMEGA_2_TAU : Subsystem
  Omega SAT : Subsystem
  TAU_2_OMEGA : Subsystem
  TAU_PD : Scope  NumInputPorts=4
  TAU_W : Scope  NumInputPorts=4
  WSATURATION : Scope  NumInputPorts=4
  XYZ POSITION : Subsystem
  w1234 : Scope  NumInputPorts=4
  w_minute : Scope  NumInputPorts=4
  w_minute1 : Scope  NumInputPorts=4
  оборотов/мин : Gain  Gain=60/(2*pi)
  оборотов/мин1 : Gain  Gain=60/(2*pi)
  x : Outport
  y : Outport  Port=2
  z : Outport  Port=3
  phi : Outport  Port=4
  theta : Outport  Port=5
  psi : Outport  Port=6
  wires:
  CONTROLLER/1(T) -> [T]
  CONTROLLER/2(tau_phi) -> [tau_phi]
  CONTROLLER/3(tau_theta) -> [tau_theta]
  CONTROLLER/4(tau_psi) -> [tau_psi]
  [T] -> TAU_2_OMEGA/1(T)
  [tau_phi] -> TAU_2_OMEGA/2(tau_phi)
  [tau_theta] -> TAU_2_OMEGA/3(tau_theta)
  [tau_psi] -> TAU_2_OMEGA/4(tau_psi)
  TAU_2_OMEGA/1(w1) -> [w1]
  TAU_2_OMEGA/2(w2) -> [w2]
  TAU_2_OMEGA/3(w3) -> [w3]
  TAU_2_OMEGA/4(w4) -> [w4]
  [w1S] -> OMEGA_2_TAU/1(w1)
  [w2S] -> OMEGA_2_TAU/2(w2)
  [w3S] -> OMEGA_2_TAU/3(w3)
  [w4S] -> OMEGA_2_TAU/4(w4)
  OMEGA_2_TAU/2(T_w) -> [T_w]
  OMEGA_2_TAU/3(tau_phiW) -> [tau_phiW]
  OMEGA_2_TAU/4(tau_thetaW) -> [tau_thetaW]
  OMEGA_2_TAU/5(tau_psiW) -> [tau_psiW]
  OMEGA_2_TAU/1(wR) -> [wR]
  [wR] -> ANGLE VELOCITY PQR(wx,xy,xz)/1(wr)
  [tau_phiW] -> ANGLE VELOCITY PQR(wx,xy,xz)/2(tau_phi)
  [tau_thetaW] -> ANGLE VELOCITY PQR(wx,xy,xz)/3(tau_theta)
  [tau_psiW] -> ANGLE VELOCITY PQR(wx,xy,xz)/4(tau_psi)
  ANGLS/1(phi) -> [phi]
  ANGLS/2(theta) -> [theta]
  ANGLS/3(psi) -> [psi]
  ANGLS/4(dphi) -> [dphi]
  ANGLS/5(dtheta) -> [dtheta]
  ANGLS/6(dpsi) -> [dpsi]
  ANGLE VELOCITY PQR(wx,xy,xz)/1(p) -> ANGLS/1(p)
  ANGLE VELOCITY PQR(wx,xy,xz)/2(q) -> ANGLS/2(q)
  ANGLE VELOCITY PQR(wx,xy,xz)/3(r) -> ANGLS/3(r)
  [phi] -> CONTROLLER/1(phi)
  [dphi] -> CONTROLLER/2(dphi)
  [theta] -> CONTROLLER/3(theta)
  [dtheta] -> CONTROLLER/4(dtheta)
  [dpsi] -> CONTROLLER/6(dpsi)
  [psi] -> CONTROLLER/5(psi)
  [T_w] -> XYZ POSITION/1(T)
  [phi] -> XYZ POSITION/2(phi)
  [theta] -> XYZ POSITION/3(theta)
  [psi] -> XYZ POSITION/4(psi)
  XYZ POSITION/1(x) -> [x]
  XYZ POSITION/2(y) -> [y]
  XYZ POSITION/3(z) -> [z]
  [z] -> CONTROLLER/7(z)
  [x] -> x/1
  [y] -> y/1
  [z] -> z/1
  [phi] -> phi/1
  [theta] -> theta/1
  [psi] -> psi/1
  [w1] -> w1234/1  "w1"
  [w2] -> w1234/2  "w2"
  [w3] -> w1234/3  "w3"
  [w4] -> w1234/4  "w4"
  [T] -> TAU_PD/1
  [tau_phi] -> TAU_PD/2
  [tau_theta] -> TAU_PD/3
  [tau_psi] -> TAU_PD/4
  [T_w] -> TAU_W/1
  [tau_phiW] -> TAU_W/2
  [tau_thetaW] -> TAU_W/3
  [tau_psiW] -> TAU_W/4
  [w1] -> оборотов/мин/1
  [w2] -> Gain1/1
  [w3] -> Gain2/1
  [w4] -> Gain3/1
  оборотов/мин/1 -> w_minute/1  "w1"
  Gain1/1 -> w_minute/2  "w2"
  Gain2/1 -> w_minute/3  "w3"
  Gain3/1 -> w_minute/4  "w4"
  [w1] -> Omega SAT/1(w1)
  [w2] -> Omega SAT/2(w2)
  [w3] -> Omega SAT/3(w3)
  [w4] -> Omega SAT/4(w4)
  Omega SAT/1(w1S) -> [w1S]
  Omega SAT/2(w2S) -> [w2S]
  Omega SAT/3(w3S) -> [w3S]
  Omega SAT/4(w4S) -> [w4S]
  [w1S] -> WSATURATION/1  "w1S"
  [w2S] -> WSATURATION/2  "w2S"
  [w3S] -> WSATURATION/3  "w3S"
  [w4S] -> WSATURATION/4  "w4S"
  [w1S] -> оборотов/мин1/1  "w1S"
  [w2S] -> Gain4/1  "w2S"
  [w3S] -> Gain5/1  "w3S"
  [w4S] -> Gain6/1  "w4S"
  оборотов/мин1/1 -> w_minute1/1  "w1"
  Gain4/1 -> w_minute1/2  "w2"
  Gain5/1 -> w_minute1/3  "w3"
  Gain6/1 -> w_minute1/4  "w4"

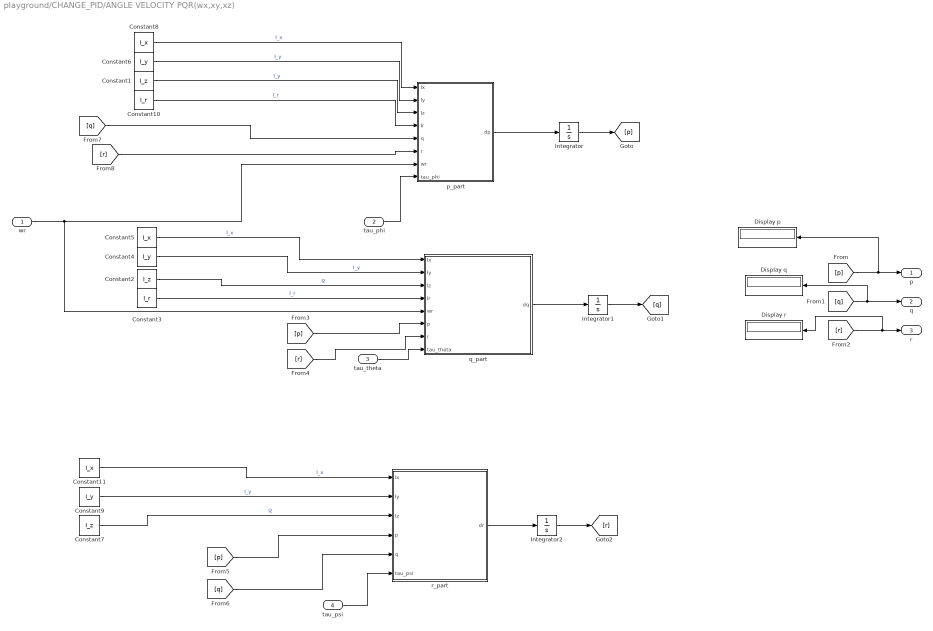
== system playground/CHANGE_PID/ANGLE VELOCITY PQR(wx,xy,xz) ==
  wr : Inport
  tau_phi : Inport  Port=2
  tau_theta : Inport  Port=3
  tau_psi : Inport  Port=4
  Constant1 : Constant  Value=I_z
  Constant10 : Constant  Value=I_r
  Constant11 : Constant  Value=I_x
  Constant2 : Constant  Value=I_z
  Constant3 : Constant  Value=I_r
  Constant4 : Constant  Value=I_y
  Constant5 : Constant  Value=I_x
  Constant6 : Constant  Value=I_y
  Constant7 : Constant  Value=I_z
  Constant8 : Constant  Value=I_x
  Constant9 : Constant  Value=I_y
  Display p : Display
  Display q : Display
  Display r : Display
  Integrator : Integrator
  Integrator1 : Integrator
  Integrator2 : Integrator
  p_part : MATLAB Function  TreatAsAtomicUnit=on
  q_part : MATLAB Function  TreatAsAtomicUnit=on
  r_part : MATLAB Function  TreatAsAtomicUnit=on
  p : Outport
  q : Outport  Port=2
  r : Outport  Port=3
  wires:
  [r] -> Display r/1, r/1
  [q] -> Display q/1, q/1
  [p] -> Display p/1, p/1
  [r] -> p_part/6(r)
  [q] -> p_part/5(q)
  [q] -> r_part/5(q)
  [p] -> r_part/4(p)
  [r] -> q_part/7(r)
  [p] -> q_part/6(p)
  Integrator2/1 -> [r]
  Integrator/1 -> [p]
  Integrator1/1 -> [q]
  r_part/1(dr) -> Integrator2/1
  q_part/1(dq) -> Integrator1/1
  p_part/1(dp) -> Integrator/1
  tau_theta/1 -> q_part/8(tau_theta)
  tau_phi/1 -> p_part/8(tau_phi)
  tau_psi/1 -> r_part/6(tau_psi)
  wr/1 -> q_part/5(wr), p_part/7(wr)
  Constant7/1 -> r_part/3(Iz)  "Iz"
  Constant9/1 -> r_part/2(Iy)  "I_y"
  Constant11/1 -> r_part/1(Ix)  "I_x"
  Constant3/1 -> q_part/4(Ir)  "I_r"
  Constant2/1 -> q_part/3(Iz)  "Iz"
  Constant4/1 -> q_part/2(Iy)  "I_y"
  Constant5/1 -> q_part/1(Ix)  "I_x"
  Constant10/1 -> p_part/4(Ir)  "I_r"
  Constant1/1 -> p_part/3(Iz)  "I_y"
  Constant6/1 -> p_part/2(Iy)  "I_y"
  Constant8/1 -> p_part/1(Ix)  "I_x"

== system playground/CHANGE_PID/ANGLS ==
  p : Inport
  q : Inport  Port=2
  r : Inport  Port=3
  Integrator : Integrator  InitialCondition=phi_init
  Integrator1 : Integrator  InitialCondition=theta_init
  Integrator2 : Integrator  InitialCondition=psi_init
  phi_part : MATLAB Function  TreatAsAtomicUnit=on
  psi_part : MATLAB Function  TreatAsAtomicUnit=on
  q1 : InportShadow  Port=2
  q2 : InportShadow  Port=2
  r1 : InportShadow  Port=3
  r2 : InportShadow  Port=3
  theta_part : MATLAB Function  TreatAsAtomicUnit=on
  phi : Outport
  theta : Outport  Port=2
  psi : Outport  Port=3
  dphi : Outport  Port=4
  dtheta : Outport  Port=5
  dpsi : Outport  Port=6
  wires:
  [phi] -> phi/1
  [theta] -> theta/1
  [psi] -> psi/1
  r2/1 -> psi_part/2(r)
  r1/1 -> theta_part/2(r)
  q2/1 -> psi_part/1(q)
  q1/1 -> theta_part/1(q)
  r/1 -> phi_part/3(r)
  q/1 -> phi_part/2(q)
  p/1 -> phi_part/1(p)
  [theta] -> phi_part/5(theta)
  [theta] -> psi_part/4(theta)
  [phi] -> psi_part/3(phi)
  [phi] -> theta_part/3(phi)
  [phi] -> phi_part/4(phi)
  Integrator2/1 -> [psi]
  psi_part/1(d_psi) -> Integrator2/1, dpsi/1
  Integrator1/1 -> [theta]
  theta_part/1(d_theta) -> Integrator1/1, dtheta/1
  Integrator/1 -> [phi]
  phi_part/1(d_phi) -> Integrator/1, dphi/1

== system playground/CHANGE_PID/CONTROLLER ==
  phi : Inport
  dphi : Inport  Port=2
  theta : Inport  Port=3
  dtheta : Inport  Port=4
  psi : Inport  Port=5
  dpsi : Inport  Port=6
  z : Inport  Port=7
  PD regulator draft : Subsystem
  PD regulator gamma1 : Subsystem
  PD regulator psi : Subsystem
  PD regulator theta : Subsystem
  T : Outport
  tau_phi : Outport  Port=2
  tau_theta : Outport  Port=3
  tau_psi : Outport  Port=4
  wires:
  PD regulator draft/1(T) -> T/1  "tau_y"
  PD regulator gamma1/1(tau_phi) -> tau_phi/1  "tau_gamma"
  PD regulator theta/1(tau_theta) -> tau_theta/1  "tau_theta"
  PD regulator psi/1(tau_psi) -> tau_psi/1  "tau_psi"
  dpsi/1 -> PD regulator psi/2((psi)')
  psi/1 -> PD regulator psi/1(psi)
  dphi/1 -> PD regulator gamma1/2((phi)')
  dtheta/1 -> PD regulator theta/2((theta)')
  theta/1 -> PD regulator theta/1(theta), PD regulator draft/2(theta)
  phi/1 -> PD regulator draft/1(phi), PD regulator gamma1/1(phi)
  z/1 -> PD regulator draft/3(z)

== system playground/CHANGE_PID/OMEGA_2_TAU ==
  w1 : Inport
  w2 : Inport  Port=2
  w3 : Inport  Port=3
  w4 : Inport  Port=4
  Constant : Constant  Value=kl*l
  Constant1 : Constant  Value=kl*l
  Constant11 : Constant  Value=kl
  Constant7 : Constant  Value=b
  Gyroscope : MATLAB Function  TreatAsAtomicUnit=on
  MATLAB Function : MATLAB Function  TreatAsAtomicUnit=on
  MATLAB Function1 : MATLAB Function  TreatAsAtomicUnit=on
  MATLAB Function2 : MATLAB Function  TreatAsAtomicUnit=on
  MATLAB Function3 : MATLAB Function  TreatAsAtomicUnit=on
  wR : Outport
  T_w : Outport  Port=2
  tau_phiW : Outport  Port=3
  tau_thetaW : Outport  Port=4
  tau_psiW : Outport  Port=5
  wires:
  Gyroscope/1(w_Gamma) -> wR/1
  MATLAB Function3/1(tau_psi) -> tau_psiW/1
  MATLAB Function2/1(tau_theta) -> tau_thetaW/1
  MATLAB Function1/1(tau_phi) -> tau_phiW/1
  MATLAB Function/1(T) -> T_w/1
  Constant11/1 -> MATLAB Function/5(k)
  Constant/1 -> MATLAB Function1/3(kl)
  Constant1/1 -> MATLAB Function2/3(kl)
  Constant7/1 -> MATLAB Function3/5(b)
  w4/1 -> MATLAB Function3/4(w4), MATLAB Function/4(w4), MATLAB Function1/2(w4), Gyroscope/4(w_4)
  w3/1 -> MATLAB Function/3(w3), MATLAB Function2/2(w3), MATLAB Function3/3(w3), Gyroscope/3(w_3)
  w2/1 -> MATLAB Function/2(w2), MATLAB Function1/1(w2), MATLAB Function3/2(w2), Gyroscope/2(w_2)
  w1/1 -> MATLAB Function/1(w1), MATLAB Function2/1(w1), MATLAB Function3/1(w1), Gyroscope/1(w_1)

== system playground/CHANGE_PID/TAU_2_OMEGA ==
  T : Inport
  tau_phi : Inport  Port=2
  tau_theta : Inport  Port=3
  tau_psi : Inport  Port=4
  Constant11 : Constant  Value=kl
  Constant12 : Constant  Value=l
  Constant7 : Constant  Value=b
  Current x{1..6} (6 alike) : Display
  MATLAB Function1 : MATLAB Function  TreatAsAtomicUnit=on
  Sqrt{1..4} (4 alike) : Sqrt
  w1 : Outport
  w2 : Outport  Port=2
  w3 : Outport  Port=3
  w4 : Outport  Port=4
  wires:
  MATLAB Function1/4(omega_4) -> Sqrt4/1
  MATLAB Function1/3(omega_3) -> Sqrt3/1
  MATLAB Function1/2(omega_2) -> Sqrt2/1
  MATLAB Function1/1(omega_1) -> Sqrt1/1
  Sqrt4/1 -> Current x1/1, w4/1  "рад/сек"
  Sqrt3/1 -> Current x2/1, w3/1  "рад/сек"
  Sqrt2/1 -> w2/1  "рад/сек"
  Sqrt1/1 -> w1/1  "рад/сек"
  tau_psi/1 -> Current x3/1, MATLAB Function1/4(tau_psi)
  tau_theta/1 -> Current x6/1, MATLAB Function1/3(tau_theta)
  tau_phi/1 -> Current x4/1, MATLAB Function1/2(tau_phi)
  T/1 -> Current x5/1, MATLAB Function1/1(T)
  Constant7/1 -> MATLAB Function1/7(b)
  Constant12/1 -> MATLAB Function1/6(l)
  Constant11/1 -> MATLAB Function1/5(k)

== system playground/CHANGE_PID/XYZ POSITION ==
  T : Inport
  phi : Inport  Port=2
  theta : Inport  Port=3
  psi : Inport  Port=4
  Constant : Constant  Value=m
  Constant1 : Constant  Value=A_x
  Constant2 : Constant  Value=A_y
  Constant3 : Constant  Value=A_z
  Integrator4 : Integrator
  XYZ : MATLAB Function  TreatAsAtomicUnit=on
  integrator1 : Integrator
  integrator2 : Integrator
  xinit : Integrator  InitialCondition=x_init
  yinit : Integrator  InitialCondition=y_init
  zinit : Integrator  InitialCondition=z_init
  x : Outport
  y : Outport  Port=2
  z : Outport  Port=3
  wires:
  zinit/1 -> z/1
  yinit/1 -> y/1
  xinit/1 -> x/1
  [dz] -> XYZ/11(dz)
  [dy] -> XYZ/10(dy)
  [dx] -> XYZ/9(dx)
  psi/1 -> XYZ/8(psi)
  theta/1 -> XYZ/7(theta)
  phi/1 -> XYZ/6(phi)
  T/1 -> XYZ/1(T)
  Constant/1 -> XYZ/2(m)
  Constant1/1 -> XYZ/3(Ax)
  XYZ/3(ddz) -> Integrator4/1
  XYZ/1(ddx) -> integrator1/1
  XYZ/2(ddy) -> integrator2/1
  Integrator4/1 -> zinit/1, [dz]
  integrator2/1 -> yinit/1, [dy]
  integrator1/1 -> xinit/1, [dx]
  Constant2/1 -> XYZ/4(Ay)
  Constant3/1 -> XYZ/5(Az)

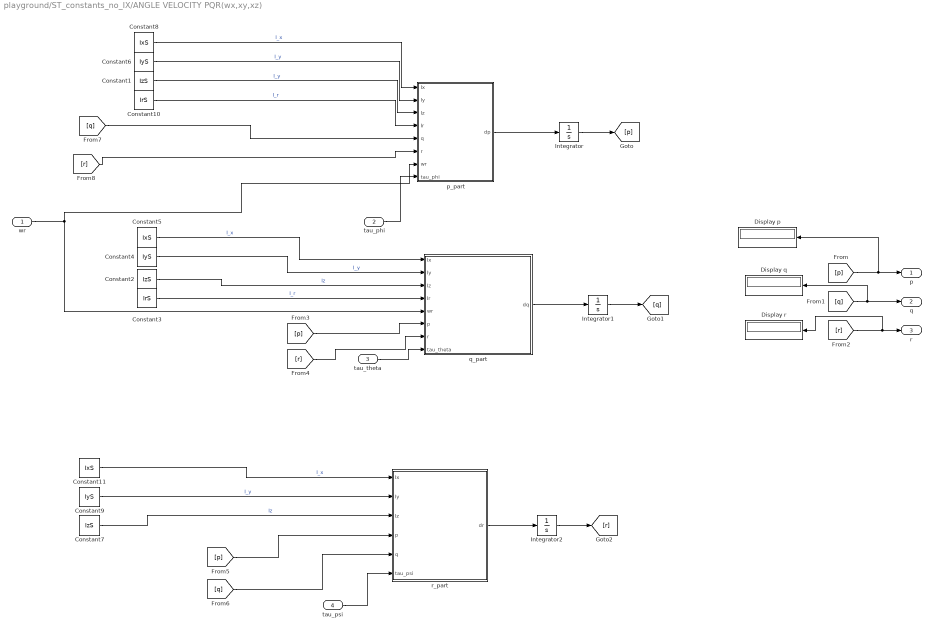
== system playground/ST_constants_no_IX/ANGLE VELOCITY PQR(wx,xy,xz) ==
  wr : Inport
  tau_phi : Inport  Port=2
  tau_theta : Inport  Port=3
  tau_psi : Inport  Port=4
  Constant1 : Constant  Value=IzS
  Constant10 : Constant  Value=IrS
  Constant11 : Constant  Value=IxS
  Constant2 : Constant  Value=IzS
  Constant3 : Constant  Value=IrS
  Constant4 : Constant  Value=IyS
  Constant5 : Constant  Value=IxS
  Constant6 : Constant  Value=IyS
  Constant7 : Constant  Value=IzS
  Constant8 : Constant  Value=IxS
  Constant9 : Constant  Value=IyS
  Display p : Display
  Display q : Display
  Display r : Display
  Integrator : Integrator
  Integrator1 : Integrator
  Integrator2 : Integrator
  p_part : MATLAB Function  TreatAsAtomicUnit=on
  q_part : MATLAB Function  TreatAsAtomicUnit=on
  r_part : MATLAB Function  TreatAsAtomicUnit=on
  p : Outport
  q : Outport  Port=2
  r : Outport  Port=3
  wires:
  [r] -> Display r/1, r/1
  [q] -> Display q/1, q/1
  [p] -> Display p/1, p/1
  [r] -> p_part/6(r)
  [q] -> p_part/5(q)
  [q] -> r_part/5(q)
  [p] -> r_part/4(p)
  [r] -> q_part/7(r)
  [p] -> q_part/6(p)
  Integrator2/1 -> [r]
  Integrator/1 -> [p]
  Integrator1/1 -> [q]
  r_part/1(dr) -> Integrator2/1
  q_part/1(dq) -> Integrator1/1
  p_part/1(dp) -> Integrator/1
  tau_theta/1 -> q_part/8(tau_theta)
  tau_phi/1 -> p_part/8(tau_phi)
  tau_psi/1 -> r_part/6(tau_psi)
  wr/1 -> q_part/5(wr), p_part/7(wr)
  Constant7/1 -> r_part/3(Iz)  "Iz"
  Constant9/1 -> r_part/2(Iy)  "I_y"
  Constant11/1 -> r_part/1(Ix)  "I_x"
  Constant3/1 -> q_part/4(Ir)  "I_r"
  Constant2/1 -> q_part/3(Iz)  "Iz"
  Constant4/1 -> q_part/2(Iy)  "I_y"
  Constant5/1 -> q_part/1(Ix)  "I_x"
  Constant10/1 -> p_part/4(Ir)  "I_r"
  Constant1/1 -> p_part/3(Iz)  "I_y"
  Constant6/1 -> p_part/2(Iy)  "I_y"
  Constant8/1 -> p_part/1(Ix)  "I_x"

== system playground/ST_constants_no_IX/ANGLS ==
  p : Inport
  q : Inport  Port=2
  r : Inport  Port=3
  Current z : Display
  Integrator : Integrator  InitialCondition=phi_iS
  Integrator1 : Integrator  InitialCondition=theta_iS
  Integrator2 : Integrator  InitialCondition=psi_iS
  phi_part : MATLAB Function  TreatAsAtomicUnit=on
  psi_part : MATLAB Function  TreatAsAtomicUnit=on
  q1 : InportShadow  Port=2
  q2 : InportShadow  Port=2
  r1 : InportShadow  Port=3
  r2 : InportShadow  Port=3
  theta_part : MATLAB Function  TreatAsAtomicUnit=on
  phi : Outport
  theta : Outport  Port=2
  psi : Outport  Port=3
  dphi : Outport  Port=4
  dtheta : Outport  Port=5
  dpsi : Outport  Port=6
  wires:
  [phi] -> phi/1
  [theta] -> theta/1
  [psi] -> psi/1
  r2/1 -> psi_part/2(r)
  r1/1 -> theta_part/2(r)
  q2/1 -> psi_part/1(q)
  q1/1 -> theta_part/1(q)
  r/1 -> phi_part/3(r)
  q/1 -> phi_part/2(q)
  p/1 -> phi_part/1(p)
  [theta] -> phi_part/5(theta)
  [theta] -> psi_part/4(theta)
  [phi] -> psi_part/3(phi)
  [phi] -> theta_part/3(phi)
  [phi] -> phi_part/4(phi)
  Integrator2/1 -> [psi]
  psi_part/1(d_psi) -> Integrator2/1, dpsi/1
  Integrator1/1 -> [theta]
  theta_part/1(d_theta) -> Integrator1/1, dtheta/1
  Integrator/1 -> [phi], Current z/1
  phi_part/1(d_phi) -> Integrator/1, dphi/1

== system playground/ST_constants_no_IX/CONTROLLER ==
  phi : Inport
  dphi : Inport  Port=2
  theta : Inport  Port=3
  dtheta : Inport  Port=4
  psi : Inport  Port=5
  dpsi : Inport  Port=6
  z : Inport  Port=7
  Current z : Display
  Current z1 : Display
  Current z2 : Display
  PD regulator draft : Subsystem
  PD regulator gamma1 : Subsystem
  PD regulator psi : Subsystem
  PD regulator theta : Subsystem
  T : Outport
  tau_phi : Outport  Port=2
  tau_theta : Outport  Port=3
  tau_psi : Outport  Port=4
  wires:
  PD regulator draft/1(T) -> T/1, Current z/1  "tau_y"
  PD regulator gamma1/1(tau_phi) -> tau_phi/1, Current z1/1  "tau_gamma"
  PD regulator theta/1(tau_theta) -> tau_theta/1  "tau_theta"
  PD regulator psi/1(tau_psi) -> tau_psi/1, Current z2/1  "tau_psi"
  dpsi/1 -> PD regulator psi/2((psi)')
  psi/1 -> PD regulator psi/1(psi)
  dphi/1 -> PD regulator gamma1/2((phi)')
  dtheta/1 -> PD regulator theta/2((theta)')
  theta/1 -> PD regulator theta/1(theta), PD regulator draft/2(theta)
  phi/1 -> PD regulator draft/1(phi), PD regulator gamma1/1(phi)
  z/1 -> PD regulator draft/3(z)

== system playground/ST_constants_no_IX/OMEGA_2_TAU ==
  w1 : Inport
  w2 : Inport  Port=2
  w3 : Inport  Port=3
  w4 : Inport  Port=4
  Constant : Constant  Value=kl*l
  Constant1 : Constant  Value=kl*l
  Constant11 : Constant  Value=kl
  Constant7 : Constant  Value=a_rS
  Current z : Display
  Current z1 : Display
  Gyroscope : MATLAB Function  TreatAsAtomicUnit=on
  MATLAB Function : MATLAB Function  TreatAsAtomicUnit=on
  MATLAB Function1 : MATLAB Function  TreatAsAtomicUnit=on
  MATLAB Function2 : MATLAB Function  TreatAsAtomicUnit=on
  MATLAB Function3 : MATLAB Function  TreatAsAtomicUnit=on
  wR : Outport
  T_w : Outport  Port=2
  tau_phiW : Outport  Port=3
  tau_thetaW : Outport  Port=4
  tau_psiW : Outport  Port=5
  wires:
  Gyroscope/1(w_Gamma) -> wR/1
  MATLAB Function3/1(tau_psi) -> tau_psiW/1
  MATLAB Function2/1(tau_theta) -> tau_thetaW/1
  MATLAB Function1/1(tau_phi) -> tau_phiW/1, Current z1/1
  MATLAB Function/1(T) -> T_w/1, Current z/1
  Constant11/1 -> MATLAB Function/5(k)
  Constant/1 -> MATLAB Function1/3(kl)
  Constant1/1 -> MATLAB Function2/3(kl)
  Constant7/1 -> MATLAB Function3/5(b)
  w4/1 -> MATLAB Function3/4(w4), MATLAB Function/4(w4), MATLAB Function1/2(w4), Gyroscope/4(w_4)
  w3/1 -> MATLAB Function/3(w3), MATLAB Function2/2(w3), MATLAB Function3/3(w3), Gyroscope/3(w_3)
  w2/1 -> MATLAB Function/2(w2), MATLAB Function1/1(w2), MATLAB Function3/2(w2), Gyroscope/2(w_2)
  w1/1 -> MATLAB Function/1(w1), MATLAB Function2/1(w1), MATLAB Function3/1(w1), Gyroscope/1(w_1)

== system playground/ST_constants_no_IX/TAU_2_OMEGA ==
  T : Inport
  tau_phi : Inport  Port=2
  tau_theta : Inport  Port=3
  tau_psi : Inport  Port=4
  Constant11 : Constant  Value=kl
  Constant12 : Constant  Value=l
  Constant7 : Constant  Value=a_rS
  Current z{,1..7} (8 alike) : Display
  MATLAB Function1 : MATLAB Function  TreatAsAtomicUnit=on
  Scope : Scope
  Sqrt{1..4} (4 alike) : Sqrt
  w1 : Outport
  w2 : Outport  Port=2
  w3 : Outport  Port=3
  w4 : Outport  Port=4
  wires:
  MATLAB Function1/4(omega_4) -> Sqrt4/1
  MATLAB Function1/3(omega_3) -> Sqrt3/1
  MATLAB Function1/2(omega_2) -> Sqrt2/1, Current z7/1
  MATLAB Function1/1(omega_1) -> Sqrt1/1
  Sqrt4/1 -> w4/1, Current z1/1  "рад/сек"
  Sqrt3/1 -> w3/1, Current z2/1  "рад/сек"
  Sqrt2/1 -> w2/1, Current z3/1  "рад/сек"
  Sqrt1/1 -> w1/1, Current z/1  "рад/сек"
  tau_psi/1 -> MATLAB Function1/4(tau_psi), Current z6/1, Scope/1
  tau_theta/1 -> MATLAB Function1/3(tau_theta)
  tau_phi/1 -> MATLAB Function1/2(tau_phi), Current z5/1
  T/1 -> MATLAB Function1/1(T), Current z4/1
  Constant7/1 -> MATLAB Function1/7(b)
  Constant12/1 -> MATLAB Function1/6(l)
  Constant11/1 -> MATLAB Function1/5(k)

== system playground/ST_constants_no_IX/XYZ POSITION ==
  T : Inport
  phi : Inport  Port=2
  theta : Inport  Port=3
  psi : Inport  Port=4
  Constant : Constant  Value=mS
  Constant1 : Constant  Value=A_x
  Constant2 : Constant  Value=A_y
  Constant3 : Constant  Value=A_z
  Integrator4 : Integrator
  XYZ : MATLAB Function  TreatAsAtomicUnit=on
  integrator1 : Integrator
  integrator2 : Integrator
  xinit : Integrator  InitialCondition=x_iS
  yinit : Integrator  InitialCondition=y_iS
  zinit : Integrator  InitialCondition=z_iS
  x : Outport
  y : Outport  Port=2
  z : Outport  Port=3
  wires:
  zinit/1 -> z/1
  yinit/1 -> y/1
  xinit/1 -> x/1
  [dz] -> XYZ/11(dz)
  [dy] -> XYZ/10(dy)
  [dx] -> XYZ/9(dx)
  psi/1 -> XYZ/8(psi)
  theta/1 -> XYZ/7(theta)
  phi/1 -> XYZ/6(phi)
  T/1 -> XYZ/1(T)
  Constant/1 -> XYZ/2(m)
  Constant1/1 -> XYZ/3(Ax)
  XYZ/3(ddz) -> Integrator4/1
  XYZ/1(ddx) -> integrator1/1
  XYZ/2(ddy) -> integrator2/1
  Integrator4/1 -> zinit/1, [dz]
  integrator2/1 -> yinit/1, [dy]
  integrator1/1 -> xinit/1, [dx]
  Constant2/1 -> XYZ/4(Ay)
  Constant3/1 -> XYZ/5(Az)

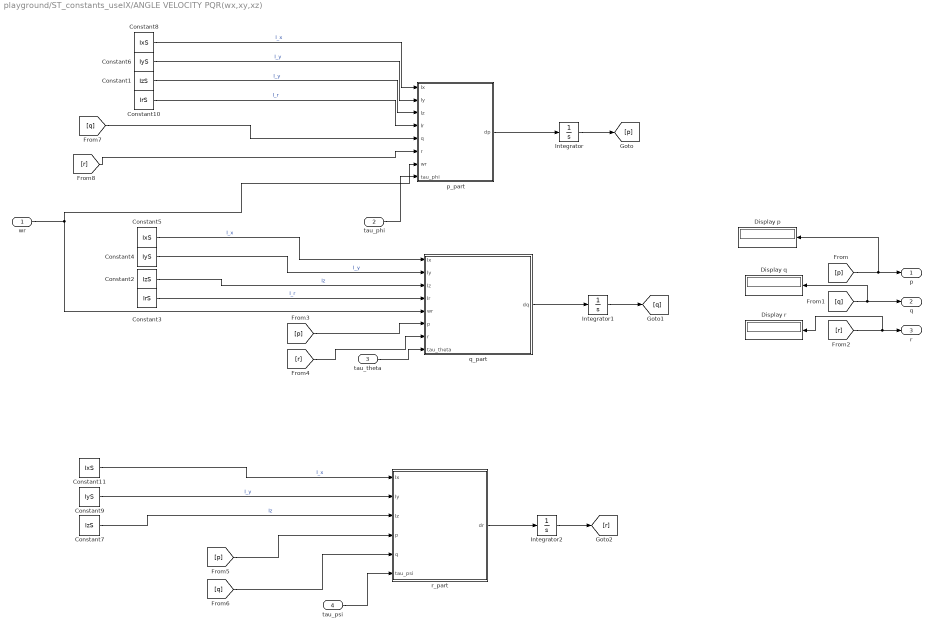
== system playground/ST_constants_useIX/ANGLE VELOCITY PQR(wx,xy,xz) ==
  wr : Inport
  tau_phi : Inport  Port=2
  tau_theta : Inport  Port=3
  tau_psi : Inport  Port=4
  Constant1 : Constant  Value=IzS
  Constant10 : Constant  Value=IrS
  Constant11 : Constant  Value=IxS
  Constant2 : Constant  Value=IzS
  Constant3 : Constant  Value=IrS
  Constant4 : Constant  Value=IyS
  Constant5 : Constant  Value=IxS
  Constant6 : Constant  Value=IyS
  Constant7 : Constant  Value=IzS
  Constant8 : Constant  Value=IxS
  Constant9 : Constant  Value=IyS
  Display p : Display
  Display q : Display
  Display r : Display
  Integrator : Integrator
  Integrator1 : Integrator
  Integrator2 : Integrator
  p_part : MATLAB Function  TreatAsAtomicUnit=on
  q_part : MATLAB Function  TreatAsAtomicUnit=on
  r_part : MATLAB Function  TreatAsAtomicUnit=on
  p : Outport
  q : Outport  Port=2
  r : Outport  Port=3
  wires:
  Constant8/1 -> p_part/1(Ix)  "I_x"
  Constant6/1 -> p_part/2(Iy)  "I_y"
  Constant1/1 -> p_part/3(Iz)  "I_y"
  Constant10/1 -> p_part/4(Ir)  "I_r"
  Constant5/1 -> q_part/1(Ix)  "I_x"
  Constant4/1 -> q_part/2(Iy)  "I_y"
  Constant2/1 -> q_part/3(Iz)  "Iz"
  Constant3/1 -> q_part/4(Ir)  "I_r"
  Constant11/1 -> r_part/1(Ix)  "I_x"
  Constant9/1 -> r_part/2(Iy)  "I_y"
  Constant7/1 -> r_part/3(Iz)  "Iz"
  wr/1 -> p_part/7(wr), q_part/5(wr)
  tau_psi/1 -> r_part/6(tau_psi)
  tau_phi/1 -> p_part/8(tau_phi)
  tau_theta/1 -> q_part/8(tau_theta)
  p_part/1(dp) -> Integrator/1
  q_part/1(dq) -> Integrator1/1
  r_part/1(dr) -> Integrator2/1
  Integrator1/1 -> [q]
  Integrator/1 -> [p]
  Integrator2/1 -> [r]
  [p] -> q_part/6(p)
  [r] -> q_part/7(r)
  [p] -> r_part/4(p)
  [q] -> r_part/5(q)
  [q] -> p_part/5(q)
  [r] -> p_part/6(r)
  [p] -> p/1, Display p/1
  [q] -> q/1, Display q/1
  [r] -> r/1, Display r/1

== system playground/ST_constants_useIX/ANGLS ==
  p : Inport
  q : Inport  Port=2
  r : Inport  Port=3
  Current z : Display
  Integrator : Integrator  InitialCondition=phi_iS
  Integrator1 : Integrator  InitialCondition=theta_iS
  Integrator2 : Integrator  InitialCondition=psi_iS
  phi_part : MATLAB Function  TreatAsAtomicUnit=on
  psi_part : MATLAB Function  TreatAsAtomicUnit=on
  q1 : InportShadow  Port=2
  q2 : InportShadow  Port=2
  r1 : InportShadow  Port=3
  r2 : InportShadow  Port=3
  theta_part : MATLAB Function  TreatAsAtomicUnit=on
  phi : Outport
  theta : Outport  Port=2
  psi : Outport  Port=3
  dphi : Outport  Port=4
  dtheta : Outport  Port=5
  dpsi : Outport  Port=6
  wires:
  phi_part/1(d_phi) -> dphi/1, Integrator/1
  Integrator/1 -> Current z/1, [phi]
  theta_part/1(d_theta) -> dtheta/1, Integrator1/1
  Integrator1/1 -> [theta]
  psi_part/1(d_psi) -> dpsi/1, Integrator2/1
  Integrator2/1 -> [psi]
  [phi] -> phi_part/4(phi)
  [phi] -> theta_part/3(phi)
  [phi] -> psi_part/3(phi)
  [theta] -> psi_part/4(theta)
  [theta] -> phi_part/5(theta)
  p/1 -> phi_part/1(p)
  q/1 -> phi_part/2(q)
  r/1 -> phi_part/3(r)
  q1/1 -> theta_part/1(q)
  q2/1 -> psi_part/1(q)
  r1/1 -> theta_part/2(r)
  r2/1 -> psi_part/2(r)
  [psi] -> psi/1
  [theta] -> theta/1
  [phi] -> phi/1

== system playground/ST_constants_useIX/CONTROLLER ==
  phi : Inport
  dphi : Inport  Port=2
  theta : Inport  Port=3
  dtheta : Inport  Port=4
  psi : Inport  Port=5
  dpsi : Inport  Port=6
  z : Inport  Port=7
  Current z : Display
  Current z1 : Display
  Current z2 : Display
  PD regulator draft : Subsystem
  PD regulator gamma1 : Subsystem
  PD regulator psi : Subsystem
  PD regulator theta : Subsystem
  T : Outport
  tau_phi : Outport  Port=2
  tau_theta : Outport  Port=3
  tau_psi : Outport  Port=4
  wires:
  z/1 -> PD regulator draft/3(z)
  phi/1 -> PD regulator gamma1/1(phi), PD regulator draft/1(phi)
  theta/1 -> PD regulator draft/2(theta), PD regulator theta/1(theta)
  dtheta/1 -> PD regulator theta/2((theta)')
  dphi/1 -> PD regulator gamma1/2((phi)')
  psi/1 -> PD regulator psi/1(psi)
  dpsi/1 -> PD regulator psi/2((psi)')
  PD regulator psi/1(tau_psi) -> Current z2/1, tau_psi/1  "tau_psi"
  PD regulator theta/1(tau_theta) -> tau_theta/1  "tau_theta"
  PD regulator gamma1/1(tau_phi) -> Current z1/1, tau_phi/1  "tau_gamma"
  PD regulator draft/1(T) -> Current z/1, T/1  "tau_y"
